simulink model "Model"  (R2023b)
settings: Solver=FixedStepAuto  StartTime=0.0  StopTime=10  FixedStep=0.002  RelTol=1e-3
model workspace (MAT data in the model file):
  a = 0
undefined symbols (not defined in the file or in its folder): X, Y, Z
libraries: sm_lib x84, nesl_utility x29, slpidlib x9, simulink x6
(part 1 of 7)
settings Model: Creator=Mas  LastModifiedBy=Mas

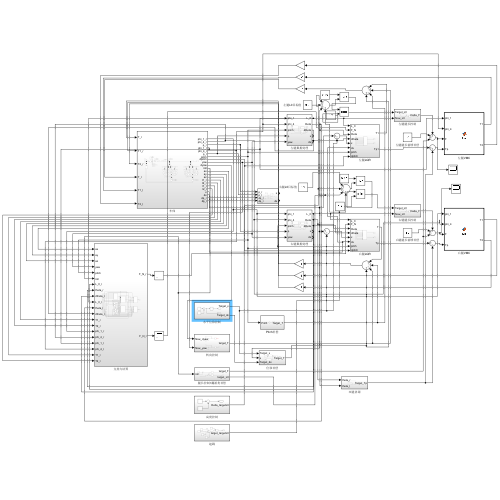
[thumbnail: Simulink's stored preview of the top-level diagram]
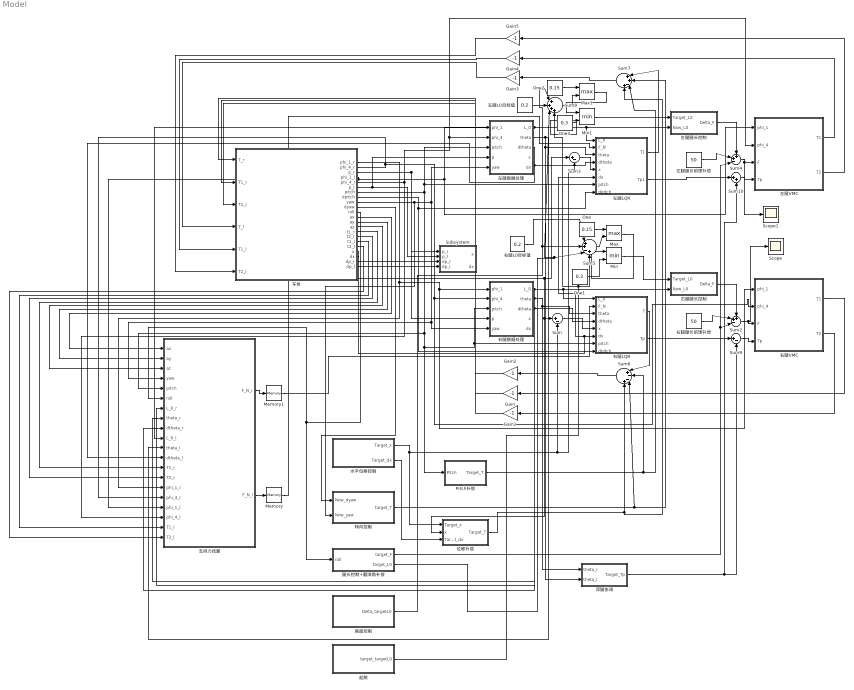
== system Model ==
  Gain{,1..5} (6 alike) : Gain  Gain=-1
  Max : MinMax  Function=max  Inputs=2
  Max1 : MinMax  Function=max  Inputs=2
  Memory : Memory
  Memory1 : Memory
  Min : MinMax  Inputs=2
  Min1 : MinMax  Inputs=2
  One : Constant  Value=0.15  OutDataTypeStr=Inherit: Inherit via back propagation
  One1 : Constant  Value=0.3  OutDataTypeStr=Inherit: Inherit via back propagation
  One2 : Constant  Value=0.15  OutDataTypeStr=Inherit: Inherit via back propagation
  One3 : Constant  Value=0.3  OutDataTypeStr=Inherit: Inherit via back propagation
  Pitch补偿 : Subsystem
  Scope : Scope
  Scope1 : Scope
  Subsystem : Subsystem
  Sum : Sum  Inputs=|+-
  Sum10 : Sum  Inputs=|++
  Sum2 : Sum  Inputs=++-|
  Sum3 : Sum  Inputs=|+-
  Sum4 : Sum  Inputs=++-|
  Sum5 : Sum  Inputs=|++-+
  Sum6 : Sum  Inputs=|+--+
  Sum7 : Sum  Inputs=|++-+
  Sum8 : Sum  Inputs=|++++
  Sum9 : Sum  Inputs=|+-
  位移补偿 : Subsystem
  双腿协调 : Subsystem
  右腿L0目标值 : Constant  Value=0.2  OutDataTypeStr=Inherit: Inherit via back propagation
  右腿LQR : Subsystem
  右腿VMC : MATLAB Function  TreatAsAtomicUnit=on
  右腿数据处理 : Subsystem
  右腿腿长前馈补偿 : Constant  Value=50  OutDataTypeStr=Inherit: Inherit via back propagation
  右腿腿长控制 : Subsystem
  左腿L0目标值 : Constant  Value=0.2  OutDataTypeStr=Inherit: Inherit via back propagation
  左腿LQR : Subsystem
  左腿VMC : MATLAB Function  TreatAsAtomicUnit=on
  左腿数据处理 : Subsystem
  左腿腿长前馈补偿 : Constant  Value=50  OutDataTypeStr=Inherit: Inherit via back propagation
  左腿腿长控制 : Subsystem
  支持力结算 : Subsystem
  水平位移控制 : Subsystem
  腿长控制+翻滚角补偿 : Subsystem
  起跳 : Subsystem
  车体 : Subsystem
  转向控制 : Subsystem
  高度控制 : Subsystem
  wires:
  右腿VMC/2(T2) -> Gain1/1
  右腿VMC/1(T1) -> Gain/1
  Sum/1 -> 右腿LQR/5(x)
  右腿腿长前馈补偿/1 -> Sum2/2
  右腿腿长控制/1(Delta_F) -> Sum2/1
  Sum2/1 -> Scope/1, 右腿VMC/3(F)
  右腿数据处理/1(L_0) -> 支持力结算/7(L_0_r), 右腿LQR/1(L_0), 右腿腿长控制/2(Now_L0)
  右腿数据处理/3(dtheta) -> 右腿LQR/4(dtheta), 支持力结算/9(dtheta_r)
  Gain2/1 -> 车体/1(T_r)
  Gain/1 -> 车体/2(T1_r)
  Gain1/1 -> 车体/3(T2_r)
  车体/7(pitch) -> Pitch补偿/1(Pitch), 右腿数据处理/3(pitch), 右腿LQR/7(pitch), 支持力结算/5(pitch), 左腿数据处理/3(pitch), 左腿LQR/7(pitch)
  车体/8(dpitch) -> 右腿LQR/8(dpitch), 左腿LQR/8(dpitch)
  车体/1(phi_1_r) -> 右腿VMC/1(phi_1), 右腿数据处理/1(phi_1), 支持力结算/15(phi_1_r)
  车体/2(phi_4_r) -> 右腿VMC/2(phi_4), 右腿数据处理/2(phi_4), 支持力结算/16(phi_4_r)
  车体/3(p_r) -> Subsystem/1(p_r), 右腿数据处理/4(p)
  车体/4(phi_1_l) -> 左腿数据处理/1(phi_1), 左腿VMC/1(phi_1), 支持力结算/17(phi_1_l)
  车体/5(phi_4_l) -> 支持力结算/18(phi_4_l), 左腿VMC/2(phi_4), 左腿数据处理/2(phi_4)
  车体/6(p_l) -> Subsystem/2(p_l), 左腿数据处理/4(p)
  左腿数据处理/2(theta) -> 支持力结算/11(theta_l), 双腿协调/2(theta_l), 左腿LQR/3(theta)
  左腿数据处理/3(dtheta) -> 支持力结算/12(dtheta_l), 左腿LQR/4(dtheta)
  Sum3/1 -> 左腿LQR/5(x)
  左腿数据处理/1(L_0) -> 支持力结算/10(L_0_l), 左腿LQR/1(L_0), 左腿腿长控制/2(Now_L0)
  Sum4/1 -> Scope1/1, 左腿VMC/3(F)
  左腿腿长前馈补偿/1 -> Sum4/2
  左腿腿长控制/1(Delta_F) -> Sum4/1
  左腿VMC/1(T1) -> Gain4/1
  左腿VMC/2(T2) -> Gain5/1
  Gain3/1 -> 车体/4(T_l)
  Gain4/1 -> 车体/5(T1_l)
  Gain5/1 -> 车体/6(T2_l)
  水平位移控制/1(Target_x) -> 位移补偿/1(Target_x), Sum3/2, Sum/2
  右腿LQR/1(T) -> Sum6/1
  左腿LQR/1(T1) -> Sum7/1
  车体/9(yaw) -> 转向控制/2(Now_yaw), 支持力结算/4(yaw), 右腿数据处理/5(yaw), 左腿数据处理/5(yaw)
  右腿数据处理/2(theta) -> 双腿协调/1(theta_r), 右腿LQR/3(theta), 支持力结算/8(theta_r)
  右腿LQR/2(Tp) -> Sum9/1
  Sum9/1 -> 右腿VMC/4(Tp)
  Sum10/1 -> 左腿VMC/4(Tp)
  左腿LQR/2(Tp1) -> Sum10/1
  双腿协调/1(Target_Tp) -> Sum10/2, Sum9/2
  转向控制/1(target_T) -> Sum6/3, Sum7/2
  车体/10(dyaw) -> 转向控制/1(Now_dyaw)
  车体/11(roll) -> 支持力结算/6(roll), 腿长控制+翻滚角补偿/1(roll)
  左腿L0目标值/1 -> Sum8/1
  右腿L0目标值/1 -> Sum5/1
  One/1 -> Max/1
  Sum5/1 -> Max/2
  Max/1 -> Min/1
  One1/1 -> Min/2
  Min/1 -> 右腿腿长控制/1(Target_L0)
  One2/1 -> Max1/1
  Sum8/1 -> Max1/2
  Max1/1 -> Min1/1
  One3/1 -> Min1/2
  Min1/1 -> 左腿腿长控制/1(Target_L0)
  腿长控制+翻滚角补偿/2(target_L0) -> Sum5/3, Sum8/3
  腿长控制+翻滚角补偿/1(target_F) -> Sum4/3, Sum2/3
  车体/12(ax) -> 支持力结算/1(ax)
  车体/13(ay) -> 支持力结算/2(ay)
  车体/14(az) -> 支持力结算/3(az)
  车体/15(t1_r) -> 支持力结算/13(T1_r)
  车体/17(t1_l) -> 支持力结算/19(T1_l)
  车体/18(t2_l) -> 支持力结算/20(T2_l)
  支持力结算/1(F_N_r) -> Memory1/1
  支持力结算/2(F_N_l) -> Memory/1
  Memory/1 -> 左腿LQR/2(F_N)
  Memory1/1 -> 右腿LQR/2(F_N)
  高度控制/1(Delta_targetL0) -> Sum8/2, Sum5/2
  起跳/1(target_targetL0) -> Sum5/4, Sum8/4
  Sum6/1 -> Gain2/1
  Sum7/1 -> Gain3/1
  车体/21(dp_r) -> Subsystem/3(dp_r)
  车体/22(dp_l) -> Subsystem/4(dp_l)
  车体/16(t2_r) -> 支持力结算/14(T2_r)
  车体/20(dx) -> 左腿LQR/6(dx), 右腿LQR/6(dx)
  车体/19(x) -> Sum3/1, 位移补偿/2(x), Sum/1
  Pitch补偿/1(Target_T) -> Sum7/3, Sum6/2
  位移补偿/1(Target_T) -> Sum7/4, Sum6/4
  水平位移控制/2(Target_dx) -> 位移补偿/3(Target_dx)

== system Model/Pitch补偿 ==
  Pitch : Inport
  Gain6 : Gain  Gain=-1
  PID Controller : slpidlib/PID Controller  Controller=PID  Form=Parallel  TimeDomain=Continuous-time  UseExternalTs=off  SampleTime=-1  IntegratorMethod=Forward Euler  FilterMethod=Forward Euler  ControllerParametersSource=internal  P=20  I=5  UseKiTs=off  D=5  N=100  UseFilter=on  TunerSelectOption=Transfer Function Based (PID Tuner App)  InitialConditionSource=internal  InitialConditionForIntegrator=0  InitialConditionForFilter=0  DifferentiatorICPrevScaledInput=0  ExternalReset=none  TrackingMode=off  Kt=1  LimitOutput=off  SatLimitsSource=internal  UpperSaturationLimit=inf  LowerSaturationLimit=-inf  LinearizeAsGain=on  AntiWindupMode=none  Kb=1  LimitIntegrator=off  UpperIntegratorSaturationLimit=inf  LowerIntegratorSaturationLimit=-inf  POutMin=[]  POutMax=[]  IOutMin=[]  IOutMax=[]  DOutMin=[]  DOutMax=[]  NOutMin=[]  NOutMax=[]  SumOutMin=[]  SumOutMax=[]  SaturationOutMin=[]  SaturationOutMax=[]  PParamMin=[]  PParamMax=[]  IParamMin=[]  IParamMax=[]  DParamMin=[]  DParamMax=[]  NParamMin=[]  NParamMax=[]  KbParamMin=[]  KbParamMax=[]  KtParamMin=[]  KtParamMax=[]  KbOutMin=[]  KbOutMax=[]  KtOutMin=[]  KtOutMax=[]  IntegratorOutMin=[]  IntegratorOutMax=[]  FilterOutMin=[]  FilterOutMax=[]  SumI1OutMin=[]  SumI1OutMax=[]  SumI2OutMin=[]  SumI2OutMax=[]  SumI3OutMin=[]  SumI3OutMax=[]  SumI4OutMin=[]  SumI4OutMax=[]  SumDOutMin=[]  SumDOutMax=[]  DifferentiatorOutMin=[]  DifferentiatorOutMax=[]  FilterDiffOutCoefMin=[]  FilterDiffOutCoefMax=[]  ReciprocalOutMin=[]  ReciprocalOutMax=[]  SumDenOutMin=[]  SumDenOutMax=[]  SumNumOutMin=[]  SumNumOutMax=[]  DivideOutMin=[]  DivideOutMax=[]  UdiffTsProdOutMin=[]  UdiffTsProdOutMax=[]  NTsProdOutMin=[]  NTsProdOutMax=[]  UintegralTsProdOutMin=[]  UintegralTsProdOutMax=[]  UngainTsProdOutMin=[]  UngainTsProdOutMax=[]  ClampingZeroOutDataTypeStr=Inherit: Inherit via back propagation  ClampingZeroOutMin=[]  ClampingZeroOutMax=[]  FilterDenConstantOutDataTypeStr=Inherit: Inherit via back propagation  FilterDenConstantOutMin=[]  FilterDenConstantOutMax=[]  PCopyOutDataTypeStr=Inherit: Inherit via back propagation  PCopyOutMin=[]  PCopyOutMax=[]  NCopyOutDataTypeStr=Inherit: Inherit via back propagation  NCopyOutMin=[]  NCopyOutMax=[]  IntegratorContinuousStateAttributes=''  IntegratorStateMustResolveToSignalObject=off  IntegratorRTWStateStorageClass=Auto  FilterContinuousStateAttributes=''  FilterStateMustResolveToSignalObject=off  FilterRTWStateStorageClass=Auto  ParallelPVariant=InternalParameters  IdealPVariant=Disabled  IVariant=InternalParameters  DVariant=InternalParameters  IntegratorVariant=Continuous  SatVariant=Disabled  AWVariant=Passthrough  PCopyVariant=Disabled  TRVariant=Disabled  FdbkBlocksVariant=Forward  IdealPFdbkVariant=Disabled  SatFdbkVariant=Disabled  DerivativeFilterVariant=ContFilter  NVariant=InternalParameters  NCopyVariant=Disabled  FilterICVariant=InternalICsFilter  IntegratorICVariant=InternalICs  ExternalResetVariant=Disabled  TRSumVariant=Passthrough  SumFdbkVariant=Disabled  SumVariant=Sum_PID  TsampFilterVariant=InternalTs  TsampNgainVariant=Passthrough  TsampIntegralVariant=Disabled_SignalSpec  ExternalSaturationOutDataTypeStr=Inherit: Same as second input
  Target_T : Outport
  wires:
  Gain6/1 -> PID Controller/1
  Pitch/1 -> Gain6/1
  PID Controller/1 -> Target_T/1

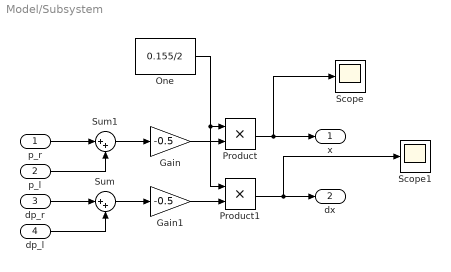
== system Model/Subsystem ==
  p_r : Inport
  p_l : Inport  Port=2
  dp_r : Inport  Port=3
  dp_l : Inport  Port=4
  Gain : Gain  Gain=-0.5
  Gain1 : Gain  Gain=-0.5
  One : Constant  Value=0.155/2  OutDataTypeStr=Inherit: Inherit via back propagation
  Product : Product
  Product1 : Product
  Scope : Scope
  Scope1 : Scope
  Sum : Sum  Inputs=|++
  Sum1 : Sum  Inputs=|++
  x : Outport
  dx : Outport  Port=2
  wires:
  dp_r/1 -> Sum/1
  dp_l/1 -> Sum/2
  p_r/1 -> Sum1/1
  p_l/1 -> Sum1/2
  Sum1/1 -> Gain/1
  Sum/1 -> Gain1/1
  Gain/1 -> Product/2
  Gain1/1 -> Product1/2
  One/1 -> Product/1, Product1/1
  Product/1 -> Scope/1, x/1
  Product1/1 -> Scope1/1, dx/1

== system Model/位移补偿 ==
  Target_x : Inport
  x : Inport  Port=2
  Target_dx : Inport  Port=3
  MATLAB Function : MATLAB Function  TreatAsAtomicUnit=on
  MATLAB Function1 : MATLAB Function  TreatAsAtomicUnit=on
  PID Controller : slpidlib/PID Controller  Controller=PID  Form=Parallel  TimeDomain=Continuous-time  UseExternalTs=off  SampleTime=-1  IntegratorMethod=Forward Euler  FilterMethod=Forward Euler  ControllerParametersSource=internal  P=2  I=3  UseKiTs=off  D=0  N=100  UseFilter=on  TunerSelectOption=Transfer Function Based (PID Tuner App)  InitialConditionSource=internal  InitialConditionForIntegrator=0  InitialConditionForFilter=0  DifferentiatorICPrevScaledInput=0  ExternalReset=none  TrackingMode=off  Kt=1  LimitOutput=off  SatLimitsSource=internal  UpperSaturationLimit=inf  LowerSaturationLimit=-inf  LinearizeAsGain=on  AntiWindupMode=none  Kb=1  LimitIntegrator=off  UpperIntegratorSaturationLimit=inf  LowerIntegratorSaturationLimit=-inf  POutMin=[]  POutMax=[]  IOutMin=[]  IOutMax=[]  DOutMin=[]  DOutMax=[]  NOutMin=[]  NOutMax=[]  SumOutMin=[]  SumOutMax=[]  SaturationOutMin=[]  SaturationOutMax=[]  PParamMin=[]  PParamMax=[]  IParamMin=[]  IParamMax=[]  DParamMin=[]  DParamMax=[]  NParamMin=[]  NParamMax=[]  KbParamMin=[]  KbParamMax=[]  KtParamMin=[]  KtParamMax=[]  KbOutMin=[]  KbOutMax=[]  KtOutMin=[]  KtOutMax=[]  IntegratorOutMin=[]  IntegratorOutMax=[]  FilterOutMin=[]  FilterOutMax=[]  SumI1OutMin=[]  SumI1OutMax=[]  SumI2OutMin=[]  SumI2OutMax=[]  SumI3OutMin=[]  SumI3OutMax=[]  SumI4OutMin=[]  SumI4OutMax=[]  SumDOutMin=[]  SumDOutMax=[]  DifferentiatorOutMin=[]  DifferentiatorOutMax=[]  FilterDiffOutCoefMin=[]  FilterDiffOutCoefMax=[]  ReciprocalOutMin=[]  ReciprocalOutMax=[]  SumDenOutMin=[]  SumDenOutMax=[]  SumNumOutMin=[]  SumNumOutMax=[]  DivideOutMin=[]  DivideOutMax=[]  UdiffTsProdOutMin=[]  UdiffTsProdOutMax=[]  NTsProdOutMin=[]  NTsProdOutMax=[]  UintegralTsProdOutMin=[]  UintegralTsProdOutMax=[]  UngainTsProdOutMin=[]  UngainTsProdOutMax=[]  ClampingZeroOutDataTypeStr=Inherit: Inherit via back propagation  ClampingZeroOutMin=[]  ClampingZeroOutMax=[]  FilterDenConstantOutDataTypeStr=Inherit: Inherit via back propagation  FilterDenConstantOutMin=[]  FilterDenConstantOutMax=[]  PCopyOutDataTypeStr=Inherit: Inherit via back propagation  PCopyOutMin=[]  PCopyOutMax=[]  NCopyOutDataTypeStr=Inherit: Inherit via back propagation  NCopyOutMin=[]  NCopyOutMax=[]  IntegratorContinuousStateAttributes=''  IntegratorStateMustResolveToSignalObject=off  IntegratorRTWStateStorageClass=Auto  FilterContinuousStateAttributes=''  FilterStateMustResolveToSignalObject=off  FilterRTWStateStorageClass=Auto  ParallelPVariant=InternalParameters  IdealPVariant=Disabled  IVariant=InternalParameters  DVariant=InternalParameters  IntegratorVariant=Continuous  SatVariant=Disabled  AWVariant=Passthrough  PCopyVariant=Disabled  TRVariant=Disabled  FdbkBlocksVariant=Forward  IdealPFdbkVariant=Disabled  SatFdbkVariant=Disabled  DerivativeFilterVariant=ContFilter  NVariant=InternalParameters  NCopyVariant=Disabled  FilterICVariant=InternalICsFilter  IntegratorICVariant=InternalICs  ExternalResetVariant=Disabled  TRSumVariant=Passthrough  SumFdbkVariant=Disabled  SumVariant=Sum_PID  TsampFilterVariant=InternalTs  TsampNgainVariant=Passthrough  TsampIntegralVariant=Disabled_SignalSpec  ExternalSaturationOutDataTypeStr=Inherit: Same as second input
  Product : Product
  Sum1 : Sum  Inputs=|+-
  Target_T : Outport
  wires:
  x/1 -> Sum1/2
  Target_x/1 -> Sum1/1
  Target_dx/1 -> MATLAB Function/1(Target_dx)
  MATLAB Function/1(Flag) -> Product/2
  Product/1 -> PID Controller/1
  PID Controller/1 -> Target_T/1
  Sum1/1 -> MATLAB Function1/1(e_0)
  MATLAB Function1/1(e) -> Product/1

== system Model/双腿协调 ==
  theta_r : Inport
  theta_l : Inport  Port=2
  PID Controller1 : slpidlib/PID Controller  Controller=PID  Form=Parallel  TimeDomain=Continuous-time  UseExternalTs=off  SampleTime=-1  IntegratorMethod=Forward Euler  FilterMethod=Forward Euler  ControllerParametersSource=internal  P=15  I=0  UseKiTs=off  D=5  N=100  UseFilter=on  TunerSelectOption=Transfer Function Based (PID Tuner App)  InitialConditionSource=internal  InitialConditionForIntegrator=0  InitialConditionForFilter=0  DifferentiatorICPrevScaledInput=0  ExternalReset=none  TrackingMode=off  Kt=1  LimitOutput=off  SatLimitsSource=internal  UpperSaturationLimit=inf  LowerSaturationLimit=-inf  LinearizeAsGain=on  AntiWindupMode=none  Kb=1  LimitIntegrator=off  UpperIntegratorSaturationLimit=inf  LowerIntegratorSaturationLimit=-inf  POutMin=[]  POutMax=[]  IOutMin=[]  IOutMax=[]  DOutMin=[]  DOutMax=[]  NOutMin=[]  NOutMax=[]  SumOutMin=[]  SumOutMax=[]  SaturationOutMin=[]  SaturationOutMax=[]  PParamMin=[]  PParamMax=[]  IParamMin=[]  IParamMax=[]  DParamMin=[]  DParamMax=[]  NParamMin=[]  NParamMax=[]  KbParamMin=[]  KbParamMax=[]  KtParamMin=[]  KtParamMax=[]  KbOutMin=[]  KbOutMax=[]  KtOutMin=[]  KtOutMax=[]  IntegratorOutMin=[]  IntegratorOutMax=[]  FilterOutMin=[]  FilterOutMax=[]  SumI1OutMin=[]  SumI1OutMax=[]  SumI2OutMin=[]  SumI2OutMax=[]  SumI3OutMin=[]  SumI3OutMax=[]  SumI4OutMin=[]  SumI4OutMax=[]  SumDOutMin=[]  SumDOutMax=[]  DifferentiatorOutMin=[]  DifferentiatorOutMax=[]  FilterDiffOutCoefMin=[]  FilterDiffOutCoefMax=[]  ReciprocalOutMin=[]  ReciprocalOutMax=[]  SumDenOutMin=[]  SumDenOutMax=[]  SumNumOutMin=[]  SumNumOutMax=[]  DivideOutMin=[]  DivideOutMax=[]  UdiffTsProdOutMin=[]  UdiffTsProdOutMax=[]  NTsProdOutMin=[]  NTsProdOutMax=[]  UintegralTsProdOutMin=[]  UintegralTsProdOutMax=[]  UngainTsProdOutMin=[]  UngainTsProdOutMax=[]  ClampingZeroOutDataTypeStr=Inherit: Inherit via back propagation  ClampingZeroOutMin=[]  ClampingZeroOutMax=[]  FilterDenConstantOutDataTypeStr=Inherit: Inherit via back propagation  FilterDenConstantOutMin=[]  FilterDenConstantOutMax=[]  PCopyOutDataTypeStr=Inherit: Inherit via back propagation  PCopyOutMin=[]  PCopyOutMax=[]  NCopyOutDataTypeStr=Inherit: Inherit via back propagation  NCopyOutMin=[]  NCopyOutMax=[]  IntegratorContinuousStateAttributes=''  IntegratorStateMustResolveToSignalObject=off  IntegratorRTWStateStorageClass=Auto  FilterContinuousStateAttributes=''  FilterStateMustResolveToSignalObject=off  FilterRTWStateStorageClass=Auto  ParallelPVariant=InternalParameters  IdealPVariant=Disabled  IVariant=InternalParameters  DVariant=InternalParameters  IntegratorVariant=Continuous  SatVariant=Disabled  AWVariant=Passthrough  PCopyVariant=Disabled  TRVariant=Disabled  FdbkBlocksVariant=Forward  IdealPFdbkVariant=Disabled  SatFdbkVariant=Disabled  DerivativeFilterVariant=ContFilter  NVariant=InternalParameters  NCopyVariant=Disabled  FilterICVariant=InternalICsFilter  IntegratorICVariant=InternalICs  ExternalResetVariant=Disabled  TRSumVariant=Passthrough  SumFdbkVariant=Disabled  SumVariant=Sum_PID  TsampFilterVariant=InternalTs  TsampNgainVariant=Passthrough  TsampIntegralVariant=Disabled_SignalSpec  ExternalSaturationOutDataTypeStr=Inherit: Same as second input
  Sum11 : Sum  Inputs=+-|
  Sum8 : Sum  Inputs=-+|
  target_Delta theta : Constant  Value=0  OutDataTypeStr=Inherit: Inherit via back propagation
  Target_Tp : Outport
  wires:
  target_Delta theta/1 -> Sum11/1
  Sum11/1 -> PID Controller1/1
  theta_l/1 -> Sum8/1
  theta_r/1 -> Sum8/2
  PID Controller1/1 -> Target_Tp/1
  Sum8/1 -> Sum11/2

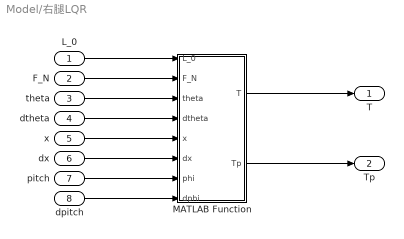
== system Model/右腿LQR ==
  L_0 : Inport
  F_N : Inport  Port=2
  theta : Inport  Port=3
  dtheta : Inport  Port=4
  x : Inport  Port=5
  dx : Inport  Port=6
  pitch : Inport  Port=7
  dpitch : Inport  Port=8
  MATLAB Function : MATLAB Function  TreatAsAtomicUnit=on
  T : Outport
  Tp : Outport  Port=2
  wires:
  dpitch/1 -> MATLAB Function/8(dphi)
  pitch/1 -> MATLAB Function/7(phi)
  dx/1 -> MATLAB Function/6(dx)
  x/1 -> MATLAB Function/5(x)
  dtheta/1 -> MATLAB Function/4(dtheta)
  theta/1 -> MATLAB Function/3(theta)
  MATLAB Function/2(Tp) -> Tp/1
  MATLAB Function/1(T) -> T/1
  L_0/1 -> MATLAB Function/1(L_0)
  F_N/1 -> MATLAB Function/2(F_N)

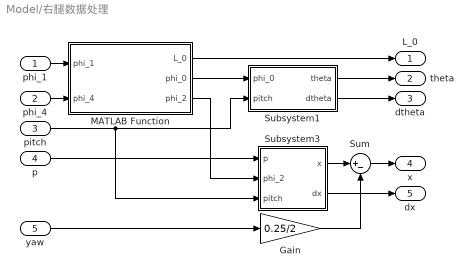
== system Model/右腿数据处理 ==
  phi_1 : Inport
  phi_4 : Inport  Port=2
  pitch : Inport  Port=3
  p : Inport  Port=4
  yaw : Inport  Port=5
  Gain : Gain  Gain=0.25/2
  MATLAB Function : MATLAB Function  TreatAsAtomicUnit=on
  Subsystem1 : Subsystem
  Subsystem3 : Subsystem
  Sum : Sum  Inputs=|+-
  L_0 : Outport
  theta : Outport  Port=2
  dtheta : Outport  Port=3
  x : Outport  Port=4
  dx : Outport  Port=5
  wires:
  Subsystem3/2(dx) -> dx/1
  MATLAB Function/2(phi_0) -> Subsystem1/1(phi_0)
  phi_1/1 -> MATLAB Function/1(phi_1)
  MATLAB Function/3(phi_2) -> Subsystem3/2(phi_2)
  Subsystem1/2(dtheta) -> dtheta/1
  MATLAB Function/1(L_0) -> L_0/1
  Subsystem1/1(theta) -> theta/1
  p/1 -> Subsystem3/1(p)
  phi_4/1 -> MATLAB Function/2(phi_4)
  pitch/1 -> Subsystem3/3(pitch), Subsystem1/2(pitch)
  Subsystem3/1(x) -> Sum/1
  Sum/1 -> x/1
  yaw/1 -> Gain/1
  Gain/1 -> Sum/2

== system Model/右腿腿长控制 ==
  Target_L0 : Inport
  Now_L0 : Inport  Port=2
  PID Controller : slpidlib/PID Controller  Controller=PID  Form=Parallel  TimeDomain=Continuous-time  UseExternalTs=off  SampleTime=-1  IntegratorMethod=Forward Euler  FilterMethod=Forward Euler  ControllerParametersSource=internal  P=750  I=10  UseKiTs=off  D=100  N=100  UseFilter=on  TunerSelectOption=Transfer Function Based (PID Tuner App)  InitialConditionSource=internal  InitialConditionForIntegrator=0  InitialConditionForFilter=0  DifferentiatorICPrevScaledInput=0  ExternalReset=none  TrackingMode=off  Kt=1  LimitOutput=off  SatLimitsSource=internal  UpperSaturationLimit=inf  LowerSaturationLimit=-inf  LinearizeAsGain=on  AntiWindupMode=none  Kb=1  LimitIntegrator=off  UpperIntegratorSaturationLimit=inf  LowerIntegratorSaturationLimit=-inf  POutMin=[]  POutMax=[]  IOutMin=[]  IOutMax=[]  DOutMin=[]  DOutMax=[]  NOutMin=[]  NOutMax=[]  SumOutMin=[]  SumOutMax=[]  SaturationOutMin=[]  SaturationOutMax=[]  PParamMin=[]  PParamMax=[]  IParamMin=[]  IParamMax=[]  DParamMin=[]  DParamMax=[]  NParamMin=[]  NParamMax=[]  KbParamMin=[]  KbParamMax=[]  KtParamMin=[]  KtParamMax=[]  KbOutMin=[]  KbOutMax=[]  KtOutMin=[]  KtOutMax=[]  IntegratorOutMin=[]  IntegratorOutMax=[]  FilterOutMin=[]  FilterOutMax=[]  SumI1OutMin=[]  SumI1OutMax=[]  SumI2OutMin=[]  SumI2OutMax=[]  SumI3OutMin=[]  SumI3OutMax=[]  SumI4OutMin=[]  SumI4OutMax=[]  SumDOutMin=[]  SumDOutMax=[]  DifferentiatorOutMin=[]  DifferentiatorOutMax=[]  FilterDiffOutCoefMin=[]  FilterDiffOutCoefMax=[]  ReciprocalOutMin=[]  ReciprocalOutMax=[]  SumDenOutMin=[]  SumDenOutMax=[]  SumNumOutMin=[]  SumNumOutMax=[]  DivideOutMin=[]  DivideOutMax=[]  UdiffTsProdOutMin=[]  UdiffTsProdOutMax=[]  NTsProdOutMin=[]  NTsProdOutMax=[]  UintegralTsProdOutMin=[]  UintegralTsProdOutMax=[]  UngainTsProdOutMin=[]  UngainTsProdOutMax=[]  ClampingZeroOutDataTypeStr=Inherit: Inherit via back propagation  ClampingZeroOutMin=[]  ClampingZeroOutMax=[]  FilterDenConstantOutDataTypeStr=Inherit: Inherit via back propagation  FilterDenConstantOutMin=[]  FilterDenConstantOutMax=[]  PCopyOutDataTypeStr=Inherit: Inherit via back propagation  PCopyOutMin=[]  PCopyOutMax=[]  NCopyOutDataTypeStr=Inherit: Inherit via back propagation  NCopyOutMin=[]  NCopyOutMax=[]  IntegratorContinuousStateAttributes=''  IntegratorStateMustResolveToSignalObject=off  IntegratorRTWStateStorageClass=Auto  FilterContinuousStateAttributes=''  FilterStateMustResolveToSignalObject=off  FilterRTWStateStorageClass=Auto  ParallelPVariant=InternalParameters  IdealPVariant=Disabled  IVariant=InternalParameters  DVariant=InternalParameters  IntegratorVariant=Continuous  SatVariant=Disabled  AWVariant=Passthrough  PCopyVariant=Disabled  TRVariant=Disabled  FdbkBlocksVariant=Forward  IdealPFdbkVariant=Disabled  SatFdbkVariant=Disabled  DerivativeFilterVariant=ContFilter  NVariant=InternalParameters  NCopyVariant=Disabled  FilterICVariant=InternalICsFilter  IntegratorICVariant=InternalICs  ExternalResetVariant=Disabled  TRSumVariant=Passthrough  SumFdbkVariant=Disabled  SumVariant=Sum_PID  TsampFilterVariant=InternalTs  TsampNgainVariant=Passthrough  TsampIntegralVariant=Disabled_SignalSpec  ExternalSaturationOutDataTypeStr=Inherit: Same as second input
  Sum1 : Sum  Inputs=+-|
  Delta_F : Outport
  wires:
  Now_L0/1 -> Sum1/2
  Sum1/1 -> PID Controller/1
  Target_L0/1 -> Sum1/1
  PID Controller/1 -> Delta_F/1

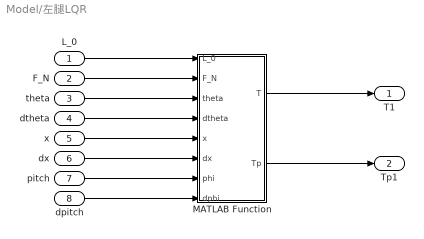
== system Model/左腿LQR ==
  L_0 : Inport
  F_N : Inport  Port=2
  theta : Inport  Port=3
  dtheta : Inport  Port=4
  x : Inport  Port=5
  dx : Inport  Port=6
  pitch : Inport  Port=7
  dpitch : Inport  Port=8
  MATLAB Function : MATLAB Function  TreatAsAtomicUnit=on
  T1 : Outport
  Tp1 : Outport  Port=2
  wires:
  MATLAB Function/2(Tp) -> Tp1/1
  MATLAB Function/1(T) -> T1/1
  dpitch/1 -> MATLAB Function/8(dphi)
  pitch/1 -> MATLAB Function/7(phi)
  dx/1 -> MATLAB Function/6(dx)
  x/1 -> MATLAB Function/5(x)
  dtheta/1 -> MATLAB Function/4(dtheta)
  theta/1 -> MATLAB Function/3(theta)
  F_N/1 -> MATLAB Function/2(F_N)
  L_0/1 -> MATLAB Function/1(L_0)

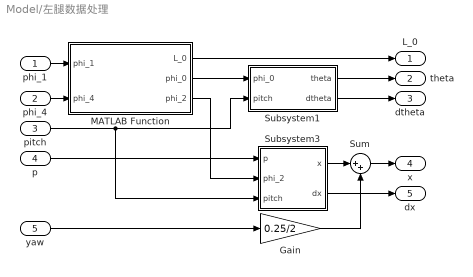
== system Model/左腿数据处理 ==
  phi_1 : Inport
  phi_4 : Inport  Port=2
  pitch : Inport  Port=3
  p : Inport  Port=4
  yaw : Inport  Port=5
  Gain : Gain  Gain=0.25/2
  MATLAB Function : MATLAB Function  TreatAsAtomicUnit=on
  Subsystem1 : Subsystem
  Subsystem3 : Subsystem
  Sum : Sum  Inputs=|++
  L_0 : Outport
  theta : Outport  Port=2
  dtheta : Outport  Port=3
  x : Outport  Port=4
  dx : Outport  Port=5
  wires:
  MATLAB Function/2(phi_0) -> Subsystem1/1(phi_0)
  phi_1/1 -> MATLAB Function/1(phi_1)
  MATLAB Function/3(phi_2) -> Subsystem3/2(phi_2)
  Subsystem1/2(dtheta) -> dtheta/1
  MATLAB Function/1(L_0) -> L_0/1
  Subsystem1/1(theta) -> theta/1
  p/1 -> Subsystem3/1(p)
  phi_4/1 -> MATLAB Function/2(phi_4)
  pitch/1 -> Subsystem3/3(pitch), Subsystem1/2(pitch)
  yaw/1 -> Gain/1
  Gain/1 -> Sum/2
  Subsystem3/1(x) -> Sum/1
  Sum/1 -> x/1
  Subsystem3/2(dx) -> dx/1

== system Model/左腿腿长控制 ==
  Target_L0 : Inport
  Now_L0 : Inport  Port=2
  PID Controller : slpidlib/PID Controller  Controller=PID  Form=Parallel  TimeDomain=Continuous-time  UseExternalTs=off  SampleTime=-1  IntegratorMethod=Forward Euler  FilterMethod=Forward Euler  ControllerParametersSource=internal  P=750  I=10  UseKiTs=off  D=100  N=100  UseFilter=on  TunerSelectOption=Transfer Function Based (PID Tuner App)  InitialConditionSource=internal  InitialConditionForIntegrator=0  InitialConditionForFilter=0  DifferentiatorICPrevScaledInput=0  ExternalReset=none  TrackingMode=off  Kt=1  LimitOutput=off  SatLimitsSource=internal  UpperSaturationLimit=inf  LowerSaturationLimit=-inf  LinearizeAsGain=on  AntiWindupMode=none  Kb=1  LimitIntegrator=off  UpperIntegratorSaturationLimit=inf  LowerIntegratorSaturationLimit=-inf  POutMin=[]  POutMax=[]  IOutMin=[]  IOutMax=[]  DOutMin=[]  DOutMax=[]  NOutMin=[]  NOutMax=[]  SumOutMin=[]  SumOutMax=[]  SaturationOutMin=[]  SaturationOutMax=[]  PParamMin=[]  PParamMax=[]  IParamMin=[]  IParamMax=[]  DParamMin=[]  DParamMax=[]  NParamMin=[]  NParamMax=[]  KbParamMin=[]  KbParamMax=[]  KtParamMin=[]  KtParamMax=[]  KbOutMin=[]  KbOutMax=[]  KtOutMin=[]  KtOutMax=[]  IntegratorOutMin=[]  IntegratorOutMax=[]  FilterOutMin=[]  FilterOutMax=[]  SumI1OutMin=[]  SumI1OutMax=[]  SumI2OutMin=[]  SumI2OutMax=[]  SumI3OutMin=[]  SumI3OutMax=[]  SumI4OutMin=[]  SumI4OutMax=[]  SumDOutMin=[]  SumDOutMax=[]  DifferentiatorOutMin=[]  DifferentiatorOutMax=[]  FilterDiffOutCoefMin=[]  FilterDiffOutCoefMax=[]  ReciprocalOutMin=[]  ReciprocalOutMax=[]  SumDenOutMin=[]  SumDenOutMax=[]  SumNumOutMin=[]  SumNumOutMax=[]  DivideOutMin=[]  DivideOutMax=[]  UdiffTsProdOutMin=[]  UdiffTsProdOutMax=[]  NTsProdOutMin=[]  NTsProdOutMax=[]  UintegralTsProdOutMin=[]  UintegralTsProdOutMax=[]  UngainTsProdOutMin=[]  UngainTsProdOutMax=[]  ClampingZeroOutDataTypeStr=Inherit: Inherit via back propagation  ClampingZeroOutMin=[]  ClampingZeroOutMax=[]  FilterDenConstantOutDataTypeStr=Inherit: Inherit via back propagation  FilterDenConstantOutMin=[]  FilterDenConstantOutMax=[]  PCopyOutDataTypeStr=Inherit: Inherit via back propagation  PCopyOutMin=[]  PCopyOutMax=[]  NCopyOutDataTypeStr=Inherit: Inherit via back propagation  NCopyOutMin=[]  NCopyOutMax=[]  IntegratorContinuousStateAttributes=''  IntegratorStateMustResolveToSignalObject=off  IntegratorRTWStateStorageClass=Auto  FilterContinuousStateAttributes=''  FilterStateMustResolveToSignalObject=off  FilterRTWStateStorageClass=Auto  ParallelPVariant=InternalParameters  IdealPVariant=Disabled  IVariant=InternalParameters  DVariant=InternalParameters  IntegratorVariant=Continuous  SatVariant=Disabled  AWVariant=Passthrough  PCopyVariant=Disabled  TRVariant=Disabled  FdbkBlocksVariant=Forward  IdealPFdbkVariant=Disabled  SatFdbkVariant=Disabled  DerivativeFilterVariant=ContFilter  NVariant=InternalParameters  NCopyVariant=Disabled  FilterICVariant=InternalICsFilter  IntegratorICVariant=InternalICs  ExternalResetVariant=Disabled  TRSumVariant=Passthrough  SumFdbkVariant=Disabled  SumVariant=Sum_PID  TsampFilterVariant=InternalTs  TsampNgainVariant=Passthrough  TsampIntegralVariant=Disabled_SignalSpec  ExternalSaturationOutDataTypeStr=Inherit: Same as second input
  Sum1 : Sum  Inputs=+-|
  Delta_F : Outport
  wires:
  Now_L0/1 -> Sum1/2
  Sum1/1 -> PID Controller/1
  Target_L0/1 -> Sum1/1
  PID Controller/1 -> Delta_F/1

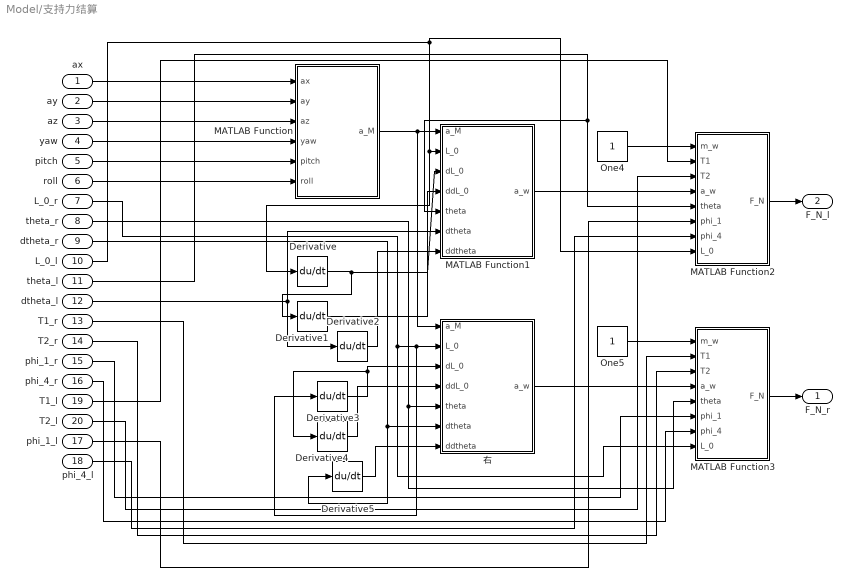
== system Model/支持力结算 ==
  ax : Inport
  ay : Inport  Port=2
  az : Inport  Port=3
  yaw : Inport  Port=4
  pitch : Inport  Port=5
  roll : Inport  Port=6
  L_0_r : Inport  Port=7
  theta_r : Inport  Port=8
  dtheta_r : Inport  Port=9
  L_0_l : Inport  Port=10
  theta_l : Inport  Port=11
  dtheta_l : Inport  Port=12
  T1_r : Inport  Port=13
  T2_r : Inport  Port=14
  phi_1_r : Inport  Port=15
  phi_4_r : Inport  Port=16
  phi_1_l : Inport  Port=17
  phi_4_l : Inport  Port=18
  T1_l : Inport  Port=19
  T2_l : Inport  Port=20
  Derivative{,1..5} (6 alike) : Derivative
  MATLAB Function : MATLAB Function  TreatAsAtomicUnit=on
  MATLAB Function1 : MATLAB Function  TreatAsAtomicUnit=on
  MATLAB Function2 : MATLAB Function  TreatAsAtomicUnit=on
  MATLAB Function3 : MATLAB Function  TreatAsAtomicUnit=on
  One4 : Constant  OutDataTypeStr=Inherit: Inherit via back propagation
  One5 : Constant  OutDataTypeStr=Inherit: Inherit via back propagation
  右 : MATLAB Function  TreatAsAtomicUnit=on
  F_N_r : Outport
  F_N_l : Outport  Port=2
  wires:
  Derivative5/1 -> 右/7(ddtheta)
  MATLAB Function1/1(a_w) -> MATLAB Function2/4(a_w)
  L_0_l/1 -> MATLAB Function2/8(L_0), Derivative/1, MATLAB Function1/2(L_0)
  MATLAB Function2/1(F_N) -> F_N_l/1
  phi_4_l/1 -> MATLAB Function2/7(phi_4)
  T2_r/1 -> MATLAB Function3/3(T2)
  MATLAB Function/1(a_M) -> 右/1(a_M), MATLAB Function1/1(a_M)
  Derivative3/1 -> 右/3(dL_0), Derivative4/1
  az/1 -> MATLAB Function/3(az)
  One4/1 -> MATLAB Function2/1(m_w)
  L_0_r/1 -> MATLAB Function3/8(L_0), Derivative3/1, 右/2(L_0)
  phi_4_r/1 -> MATLAB Function3/7(phi_4)
  dtheta_r/1 -> Derivative5/1, 右/6(dtheta)
  右/1(a_w) -> MATLAB Function3/4(a_w)
  Derivative/1 -> MATLAB Function1/3(dL_0), Derivative1/1
  dtheta_l/1 -> Derivative2/1, MATLAB Function1/6(dtheta)
  MATLAB Function3/1(F_N) -> F_N_r/1
  phi_1_l/1 -> MATLAB Function2/6(phi_1)
  Derivative2/1 -> MATLAB Function1/7(ddtheta)
  ay/1 -> MATLAB Function/2(ay)
  phi_1_r/1 -> MATLAB Function3/6(phi_1)
  theta_l/1 -> MATLAB Function2/5(theta), MATLAB Function1/5(theta)
  Derivative4/1 -> 右/4(ddL_0)
  Derivative1/1 -> MATLAB Function1/4(ddL_0)
  One5/1 -> MATLAB Function3/1(m_w)
  theta_r/1 -> MATLAB Function3/5(theta), 右/5(theta)
  pitch/1 -> MATLAB Function/5(pitch)
  T1_l/1 -> MATLAB Function2/2(T1)
  T2_l/1 -> MATLAB Function2/3(T2)
  T1_r/1 -> MATLAB Function3/2(T1)
  ax/1 -> MATLAB Function/1(ax)
  roll/1 -> MATLAB Function/6(roll)
  yaw/1 -> MATLAB Function/4(yaw)

== system Model/水平位移控制 ==
  Integrator : Integrator
  Step : Step  SampleTime=0
  Step1 : Step  Time=1.6  After=0  SampleTime=0
  Sum1 : Sum  Inputs=|+-
  Target_x : Outport
  Target_dx : Outport  Port=2
  wires:
  Step/1 -> Sum1/1
  Sum1/1 -> Target_dx/1, Integrator/1
  Step1/1 -> Sum1/2
  Integrator/1 -> Target_x/1

== system Model/腿长控制+翻滚角补偿 ==
  roll : Inport
  PID Controller : slpidlib/PID Controller  Controller=PID  Form=Parallel  TimeDomain=Continuous-time  UseExternalTs=off  SampleTime=-1  IntegratorMethod=Forward Euler  FilterMethod=Forward Euler  ControllerParametersSource=internal  P=10  I=0  UseKiTs=off  D=0  N=100  UseFilter=on  TunerSelectOption=Transfer Function Based (PID Tuner App)  InitialConditionSource=internal  InitialConditionForIntegrator=0  InitialConditionForFilter=0  DifferentiatorICPrevScaledInput=0  ExternalReset=none  TrackingMode=off  Kt=1  LimitOutput=off  SatLimitsSource=internal  UpperSaturationLimit=inf  LowerSaturationLimit=-inf  LinearizeAsGain=on  AntiWindupMode=none  Kb=1  LimitIntegrator=off  UpperIntegratorSaturationLimit=inf  LowerIntegratorSaturationLimit=-inf  POutMin=[]  POutMax=[]  IOutMin=[]  IOutMax=[]  DOutMin=[]  DOutMax=[]  NOutMin=[]  NOutMax=[]  SumOutMin=[]  SumOutMax=[]  SaturationOutMin=[]  SaturationOutMax=[]  PParamMin=[]  PParamMax=[]  IParamMin=[]  IParamMax=[]  DParamMin=[]  DParamMax=[]  NParamMin=[]  NParamMax=[]  KbParamMin=[]  KbParamMax=[]  KtParamMin=[]  KtParamMax=[]  KbOutMin=[]  KbOutMax=[]  KtOutMin=[]  KtOutMax=[]  IntegratorOutMin=[]  IntegratorOutMax=[]  FilterOutMin=[]  FilterOutMax=[]  SumI1OutMin=[]  SumI1OutMax=[]  SumI2OutMin=[]  SumI2OutMax=[]  SumI3OutMin=[]  SumI3OutMax=[]  SumI4OutMin=[]  SumI4OutMax=[]  SumDOutMin=[]  SumDOutMax=[]  DifferentiatorOutMin=[]  DifferentiatorOutMax=[]  FilterDiffOutCoefMin=[]  FilterDiffOutCoefMax=[]  ReciprocalOutMin=[]  ReciprocalOutMax=[]  SumDenOutMin=[]  SumDenOutMax=[]  SumNumOutMin=[]  SumNumOutMax=[]  DivideOutMin=[]  DivideOutMax=[]  UdiffTsProdOutMin=[]  UdiffTsProdOutMax=[]  NTsProdOutMin=[]  NTsProdOutMax=[]  UintegralTsProdOutMin=[]  UintegralTsProdOutMax=[]  UngainTsProdOutMin=[]  UngainTsProdOutMax=[]  ClampingZeroOutDataTypeStr=Inherit: Inherit via back propagation  ClampingZeroOutMin=[]  ClampingZeroOutMax=[]  FilterDenConstantOutDataTypeStr=Inherit: Inherit via back propagation  FilterDenConstantOutMin=[]  FilterDenConstantOutMax=[]  PCopyOutDataTypeStr=Inherit: Inherit via back propagation  PCopyOutMin=[]  PCopyOutMax=[]  NCopyOutDataTypeStr=Inherit: Inherit via back propagation  NCopyOutMin=[]  NCopyOutMax=[]  IntegratorContinuousStateAttributes=''  IntegratorStateMustResolveToSignalObject=off  IntegratorRTWStateStorageClass=Auto  FilterContinuousStateAttributes=''  FilterStateMustResolveToSignalObject=off  FilterRTWStateStorageClass=Auto  ParallelPVariant=InternalParameters  IdealPVariant=Disabled  IVariant=InternalParameters  DVariant=InternalParameters  IntegratorVariant=Continuous  SatVariant=Disabled  AWVariant=Passthrough  PCopyVariant=Disabled  TRVariant=Disabled  FdbkBlocksVariant=Forward  IdealPFdbkVariant=Disabled  SatFdbkVariant=Disabled  DerivativeFilterVariant=ContFilter  NVariant=InternalParameters  NCopyVariant=Disabled  FilterICVariant=InternalICsFilter  IntegratorICVariant=InternalICs  ExternalResetVariant=Disabled  TRSumVariant=Passthrough  SumFdbkVariant=Disabled  SumVariant=Sum_PID  TsampFilterVariant=InternalTs  TsampNgainVariant=Passthrough  TsampIntegralVariant=Disabled_SignalSpec  ExternalSaturationOutDataTypeStr=Inherit: Same as second input
  PID Controller1 : slpidlib/PID Controller  Controller=PID  Form=Parallel  TimeDomain=Continuous-time  UseExternalTs=off  SampleTime=-1  IntegratorMethod=Forward Euler  FilterMethod=Forward Euler  ControllerParametersSource=internal  P=2  I=0  UseKiTs=off  D=0  N=100  UseFilter=on  TunerSelectOption=Transfer Function Based (PID Tuner App)  InitialConditionSource=internal  InitialConditionForIntegrator=0  InitialConditionForFilter=0  DifferentiatorICPrevScaledInput=0  ExternalReset=none  TrackingMode=off  Kt=1  LimitOutput=off  SatLimitsSource=internal  UpperSaturationLimit=inf  LowerSaturationLimit=-inf  LinearizeAsGain=on  AntiWindupMode=none  Kb=1  LimitIntegrator=off  UpperIntegratorSaturationLimit=inf  LowerIntegratorSaturationLimit=-inf  POutMin=[]  POutMax=[]  IOutMin=[]  IOutMax=[]  DOutMin=[]  DOutMax=[]  NOutMin=[]  NOutMax=[]  SumOutMin=[]  SumOutMax=[]  SaturationOutMin=[]  SaturationOutMax=[]  PParamMin=[]  PParamMax=[]  IParamMin=[]  IParamMax=[]  DParamMin=[]  DParamMax=[]  NParamMin=[]  NParamMax=[]  KbParamMin=[]  KbParamMax=[]  KtParamMin=[]  KtParamMax=[]  KbOutMin=[]  KbOutMax=[]  KtOutMin=[]  KtOutMax=[]  IntegratorOutMin=[]  IntegratorOutMax=[]  FilterOutMin=[]  FilterOutMax=[]  SumI1OutMin=[]  SumI1OutMax=[]  SumI2OutMin=[]  SumI2OutMax=[]  SumI3OutMin=[]  SumI3OutMax=[]  SumI4OutMin=[]  SumI4OutMax=[]  SumDOutMin=[]  SumDOutMax=[]  DifferentiatorOutMin=[]  DifferentiatorOutMax=[]  FilterDiffOutCoefMin=[]  FilterDiffOutCoefMax=[]  ReciprocalOutMin=[]  ReciprocalOutMax=[]  SumDenOutMin=[]  SumDenOutMax=[]  SumNumOutMin=[]  SumNumOutMax=[]  DivideOutMin=[]  DivideOutMax=[]  UdiffTsProdOutMin=[]  UdiffTsProdOutMax=[]  NTsProdOutMin=[]  NTsProdOutMax=[]  UintegralTsProdOutMin=[]  UintegralTsProdOutMax=[]  UngainTsProdOutMin=[]  UngainTsProdOutMax=[]  ClampingZeroOutDataTypeStr=Inherit: Inherit via back propagation  ClampingZeroOutMin=[]  ClampingZeroOutMax=[]  FilterDenConstantOutDataTypeStr=Inherit: Inherit via back propagation  FilterDenConstantOutMin=[]  FilterDenConstantOutMax=[]  PCopyOutDataTypeStr=Inherit: Inherit via back propagation  PCopyOutMin=[]  PCopyOutMax=[]  NCopyOutDataTypeStr=Inherit: Inherit via back propagation  NCopyOutMin=[]  NCopyOutMax=[]  IntegratorContinuousStateAttributes=''  IntegratorStateMustResolveToSignalObject=off  IntegratorRTWStateStorageClass=Auto  FilterContinuousStateAttributes=''  FilterStateMustResolveToSignalObject=off  FilterRTWStateStorageClass=Auto  ParallelPVariant=InternalParameters  IdealPVariant=Disabled  IVariant=InternalParameters  DVariant=InternalParameters  IntegratorVariant=Continuous  SatVariant=Disabled  AWVariant=Passthrough  PCopyVariant=Disabled  TRVariant=Disabled  FdbkBlocksVariant=Forward  IdealPFdbkVariant=Disabled  SatFdbkVariant=Disabled  DerivativeFilterVariant=ContFilter  NVariant=InternalParameters  NCopyVariant=Disabled  FilterICVariant=InternalICsFilter  IntegratorICVariant=InternalICs  ExternalResetVariant=Disabled  TRSumVariant=Passthrough  SumFdbkVariant=Disabled  SumVariant=Sum_PID  TsampFilterVariant=InternalTs  TsampNgainVariant=Passthrough  TsampIntegralVariant=Disabled_SignalSpec  ExternalSaturationOutDataTypeStr=Inherit: Same as second input
  Ramp : simulink/Sources/Ramp  slope=0  start=9  InitialOutput=0
  Ramp1 : simulink/Sources/Ramp  slope=0  start=11  InitialOutput=0
  Sum1 : Sum  Inputs=+-|
  Sum11 : Sum  Inputs=|+-
  target_F : Outport
  target_L0 : Outport  Port=2
  wires:
  Sum1/1 -> PID Controller1/1, PID Controller/1
  Ramp1/1 -> Sum11/2
  roll/1 -> Sum1/2
  PID Controller/1 -> target_F/1
  Ramp/1 -> Sum11/1
  PID Controller1/1 -> target_L0/1
  Sum11/1 -> Sum1/1

== system Model/起跳 ==
  One4 : Constant  Value=0  OutDataTypeStr=Inherit: Inherit via back propagation
  Product : Product
  Step : Step  After=-0.05  SampleTime=0
  Step1 : Step  Time=2  After=0.15  SampleTime=0
  Step2 : Step  Time=2.16  After=-0.15  SampleTime=0
  Step3 : Step  Time=2.5  After=0.05  SampleTime=0
  Sum1 : Sum  Inputs=|++++
  target_targetL0 : Outport
  wires:
  Step/1 -> Sum1/1
  Sum1/1 -> Product/2
  Product/1 -> target_targetL0/1
  One4/1 -> Product/1
  Step1/1 -> Sum1/2
  Step2/1 -> Sum1/3
  Step3/1 -> Sum1/4
